simulink model "cacc"  (R2025a)
settings: Solver=VariableStepAuto  StartTime=0.0  StopTime=10.0  RelTol=1e-3
settings Model: Creator=matthewkeller  LastModifiedBy=matthewkeller

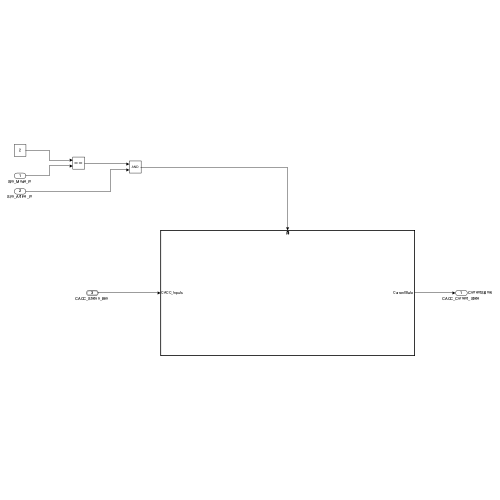
[thumbnail: Simulink's stored preview of the top-level diagram]
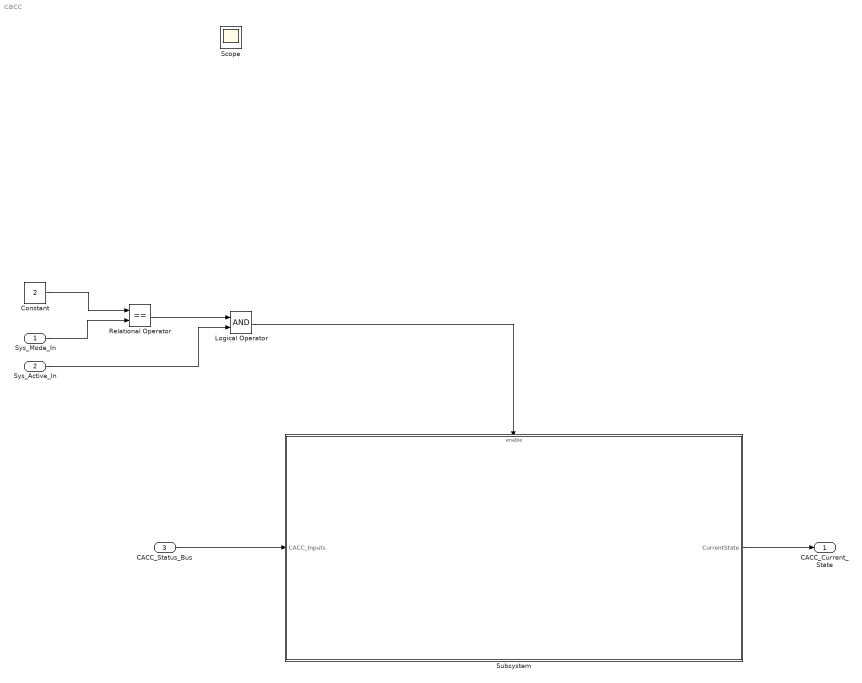
== system cacc ==
  Sys_Mode_In : Inport  OutDataTypeStr=int8
  Sys_Active_In : Inport  Port=2  OutDataTypeStr=boolean
  CACC_Status_Bus : Inport  Port=3  OutDataTypeStr=Bus: CACCStatusBus
  Constant : Constant  Value=2  OutDataTypeStr=int8
  Logical Operator : Logic  AllPortsSameDT=off  OutDataTypeStr=boolean
  Relational Operator : RelationalOperator  Operator===  OutDataTypeStr=boolean  RndMeth=Simplest  InputSameDT=off
  Subsystem : Subsystem
  CACC_Current_State : Outport  SignalName=CurrentSignal
  Scope : Scope
      settings: ActiveDisplayYMinimum=-1  ActiveDisplayYMaximum=1
  wires:
  Sys_Mode_In/1 -> Relational Operator/2
  Constant/1 -> Relational Operator/1
  Sys_Active_In/1 -> Logical Operator/2
  Relational Operator/1 -> Logical Operator/1
  CACC_Status_Bus/1 -> Subsystem/1(CACC_Inputs)
  Subsystem/1(CurrentState) -> CACC_Current_State/1
  Logical Operator/1 -> Subsystem/Enable

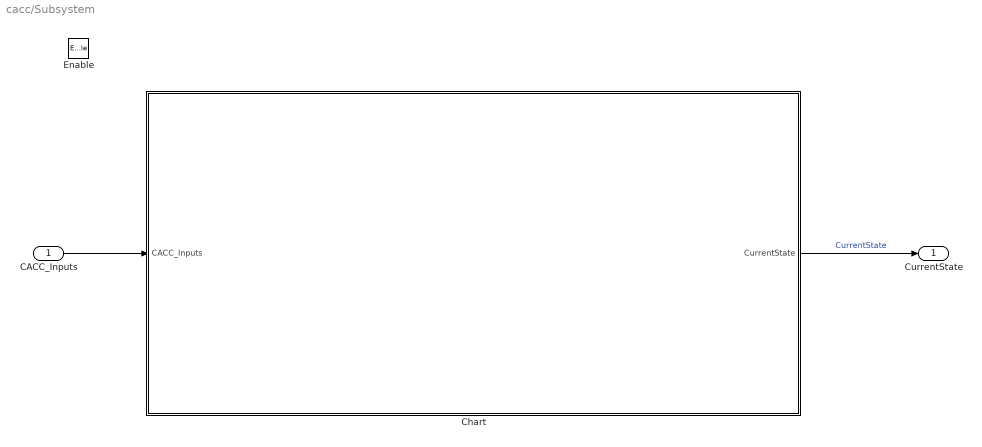
== system cacc/Subsystem ==
  CACC_Inputs : Inport
  Enable : EnablePort
  Chart : Stateflow chart  TreatAsAtomicUnit=on
  CurrentState : Outport
  wires:
  CACC_Inputs/1 -> Chart/1(CACC_Inputs)
  Chart/1(CurrentState) -> CurrentState/1  "CurrentState"

== stateflow chart cacc/Subsystem/Chart ==
  settings: executeAtInitialization=1
  state CACC_Deactivated
    entry:
    CurrentState = 0;
  state CACC_Active
    entry:
    CurrentState = 2;
  state CACC_Standby
    entry:
    CurrentState = 1;
  (default) -> CACC_Deactivated
  CACC_Active -> CACC_Deactivated [order 2] : [CACC_Inputs.Timeout_Event]
  CACC_Active -> CACC_Deactivated [order 1] : [CACC_Inputs.Cancel_Pressed || CACC_Inputs.Driver_Brakes]
  CACC_Deactivated -> CACC_Standby : [CACC_Inputs.ACC_Enable_Pressed && CACC_Inputs.V2X_Switch_ON && CACC_Inputs.Longitudinal_Switch_ON]
  CACC_Standby -> CACC_Active : [CACC_Inputs.Set_Resume && CACC_Inputs.In_CACC_Speed_Range]
  data: CACC_Inputs input Bus: CACCStatusBus; CurrentState output int8
